simulink model "ABS_Breaking_Model"  (R2018a)
settings: Solver=VariableStepAuto  StartTime=0.0  StopTime=20  RelTol=1e-3
model workspace (MATLAB code in the model file):
  | c1=1.2801;
  | c2=23.99;
  | c3=0.52;
  | ctrl=1;
  | Pbmax=1500;
  | m=50;
  | g=32.18;
  | J=5;
  | Tm=5;
  | Tb=0.01;
  | Rr=1.25;
  | Fz=3;
  | Kf=1;
  | V0=88;
  | slip=[0 0.05 0.1 0.15 0.2 0.25 0.3 0.35 0.4 0.45 0.5 0.55 0.6 0.65 0.7 0.75 0.8 0.85 0.9 0.95 1];
  | mu=[0 0.4 0.8 0.97 1 0.98 0.96 0.94 0.92 0.9 0.88 0.855 0.83 0.81 0.79 0.77 0.75 0.73 0.72 0.71 0.7];
  | b0 = 1.6500;
  | b1 = -7.6118;
  | b2 = 1122.6;
  | b3 = -0.0073600;
  | b4 = 144.8200;
  | b5 = -0.076614;
  | b6 = -0.0038600;
  | b7 = 0.085055;
  | b8 = 0.075719;
  | b9 = 0.023655;
  | b10 = 0.023655;
settings Model: Creator=uzeyi  LastModifiedBy=uzeyi

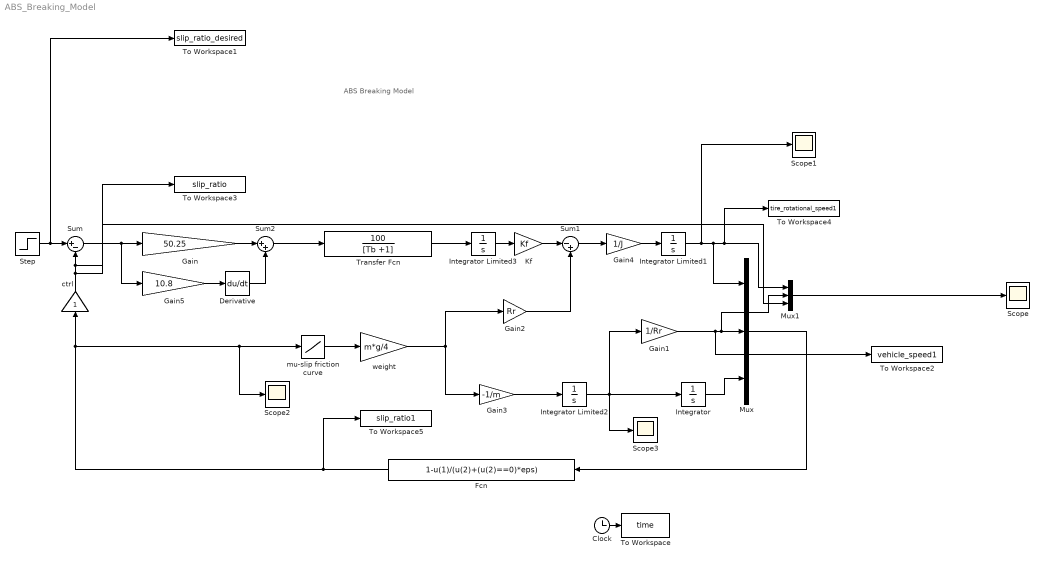
== system ABS_Breaking_Model ==
  note: ABS Breaking Model
  Clock : Clock
  Derivative : Derivative
  Fcn : Fcn  Expr=1-u(1)/(u(2)+(u(2)==0)*eps)
  Gain : Gain  Gain=50.25
  Gain1 : Gain  Gain=1/Rr
  Gain2 : Gain  Gain=Rr
  Gain3 : Gain  Gain=-1/m
  Gain4 : Gain  Gain=1/J
  Gain5 : Gain  Gain=10.8
  Integrator : Integrator
  Integrator Limited1 : Integrator  InitialCondition=V0/Rr  LimitOutput=on  UpperSaturationLimit=80  LowerSaturationLimit=0
  Integrator Limited2 : Integrator  InitialCondition=V0  LimitOutput=on  UpperSaturationLimit=1000  LowerSaturationLimit=0
  Integrator Limited3 : Integrator  LimitOutput=on  UpperSaturationLimit=Pbmax  LowerSaturationLimit=0
  Kf : Gain  Gain=Kf
  Mux : Mux  Inputs=3
  Mux1 : Mux  Inputs=3
  Scope{,1..3} (4 alike) : Scope
  Step : Step  Time=0.2  After=0.2  SampleTime=0
  Sum : Sum  Inputs=|+-
  Sum1 : Sum  Inputs=|-+
  Sum2 : Sum  Inputs=|++
  To Workspace : ToWorkspace  VariableName=time  SampleTime=-1
  To Workspace1 : ToWorkspace  VariableName=slip_ratio_desired  SampleTime=-1
  To Workspace2 : ToWorkspace  VariableName=vehicle_speed1  SampleTime=-1
  To Workspace3 : ToWorkspace  VariableName=slip_ratio  SampleTime=-1
  To Workspace4 : ToWorkspace  VariableName=tire_rotational_speed1  SampleTime=-1
  To Workspace5 : ToWorkspace  VariableName=slip_ratio1  SampleTime=-1
  Transfer Fcn : TransferFcn  Numerator=[100]  Denominator=[Tb +1]
  ctrl : Gain
  mu-slip friction curve : Lookup_n-D  NumberOfTableDimensions=1  BreakpointsForDimension1=slip  Table=mu  SaturateOnIntegerOverflow=on  InputSameDT=on
  weight : Gain  Gain=m*g/4
  wires:
  Gain1/1 -> To Workspace2/1, Mux1/2, Mux/2
  Fcn/1 -> To Workspace5/1, mu-slip friction curve/1, Scope2/1, ctrl/1
  Gain4/1 -> Integrator Limited1/1
  Integrator Limited3/1 -> Kf/1
  Sum1/1 -> Gain4/1
  weight/1 -> Gain3/1, Gain2/1
  Gain2/1 -> Sum1/2
  Mux1/1 -> Scope/1
  Mux/1 -> Fcn/1
  Transfer Fcn/1 -> Integrator Limited3/1
  Integrator/1 -> Mux/3
  Integrator Limited2/1 -> Scope3/1, Integrator/1, Gain1/1
  Kf/1 -> Sum1/1
  mu-slip friction curve/1 -> weight/1
  Gain3/1 -> Integrator Limited2/1
  Step/1 -> To Workspace1/1, Sum/1
  ctrl/1 -> Mux1/3, To Workspace3/1, Sum/2
  Integrator Limited1/1 -> Scope1/1, Mux/1, Mux1/1, To Workspace4/1
  Sum/1 -> Gain/1, Gain5/1
  Sum2/1 -> Transfer Fcn/1
  Gain/1 -> Sum2/1
  Gain5/1 -> Derivative/1
  Derivative/1 -> Sum2/2
  Clock/1 -> To Workspace/1
